simulink model "ESE4481_hw4_controls"  (R2021a)
settings: Solver=VariableStepAuto  StartTime=0.0  StopTime=10.0  RelTol=1e-3
values from neighbouring files (symbols this model uses):
  K_A = place(A_aileron, B_aileron, [-2,-4,-1])    [ESE4481_hw4_poleplacement.m]
  K_E = place(A_elevator, B_elevator, [-2,-4,-1])    [ESE4481_hw4_poleplacement.m]
  K_R = place(A_rudder, B_rudder, [-2,-4])    [ESE4481_hw4_poleplacement.m]
  K_T = place(A_throttle, B_throttle, [-2,-4])    [ESE4481_hw4_poleplacement.m]
undefined symbols (not defined in the file or in its folder): A_aileron, A_elevator, A_rudder, A_throttle, B_aileron, B_elevator, B_rudder, B_throttle, F_aileron, F_elevator, F_rudder, F_throttle
settings Model: Creator=Liza  LastModifiedBy=Liza

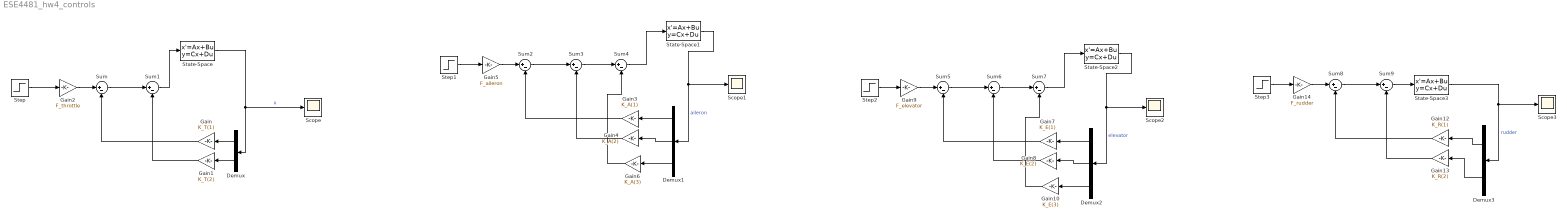
== system ESE4481_hw4_controls ==
  Demux : Demux  Outputs=2
  Demux1 : Demux  Outputs=3
  Demux2 : Demux  Outputs=3
  Demux3 : Demux  Outputs=2
  Gain : Gain  Gain=K_T(1)
  Gain1 : Gain  Gain=K_T(2)
  Gain10 : Gain  Gain=K_E(3)
  Gain12 : Gain  Gain=K_R(1)
  Gain13 : Gain  Gain=K_R(2)
  Gain14 : Gain  Gain=F_rudder
  Gain2 : Gain  Gain=F_throttle
  Gain3 : Gain  Gain=K_A(1)
  Gain4 : Gain  Gain=K_A(2)
  Gain5 : Gain  Gain=F_aileron
  Gain6 : Gain  Gain=K_A(3)
  Gain7 : Gain  Gain=K_E(1)
  Gain8 : Gain  Gain=K_E(2)
  Gain9 : Gain  Gain=F_elevator
  Scope{,1..3} (4 alike) : Scope
  State-Space : StateSpace  A=A_throttle  B=B_throttle  C=[1,0;0,1]  D=[0;0]  InitialCondition=[0,0]
  State-Space1 : StateSpace  A=A_aileron  B=B_aileron  C=[1,0,0;0,1,0;0,0,1]  D=[0;0;0]  InitialCondition=[0;0;0]
  State-Space2 : StateSpace  A=A_elevator  B=B_elevator  C=[1,0,0;0,1,0;0,0,1]  D=[0;0;0]  InitialCondition=[0;0;0]
  State-Space3 : StateSpace  A=A_rudder  B=B_rudder  C=[1,0;0,1]  D=[0;0]  InitialCondition=[0;0]
  Step : Step  Time=5  SampleTime=0
  Step1 : Step  Time=5  SampleTime=0
  Step2 : Step  Time=3  SampleTime=0
  Step3 : Step  Time=5  After=0  SampleTime=0
  Sum{,1..9} (10 alike) : Sum  Inputs=|+-
  wires:
  Sum/1 -> Sum1/1
  Sum1/1 -> State-Space/1
  State-Space/1 -> Demux/1, Scope/1  "x"
  Demux/1 -> Gain/1
  Demux/2 -> Gain1/1
  Gain1/1 -> Sum1/2
  Gain/1 -> Sum/2
  Gain2/1 -> Sum/1
  Step1/1 -> Gain5/1
  Gain4/1 -> Sum3/2
  Gain3/1 -> Sum2/2
  Demux1/2 -> Gain4/1
  Gain5/1 -> Sum2/1
  State-Space1/1 -> Demux1/1, Scope1/1  "aileron"
  Sum2/1 -> Sum3/1
  Demux1/1 -> Gain3/1
  Demux1/3 -> Gain6/1
  Sum3/1 -> Sum4/1
  Gain6/1 -> Sum4/2
  Sum4/1 -> State-Space1/1
  Sum7/1 -> State-Space2/1
  Step2/1 -> Gain9/1
  Demux2/3 -> Gain10/1
  Sum5/1 -> Sum6/1
  Gain8/1 -> Sum6/2
  Gain9/1 -> Sum5/1
  Demux2/2 -> Gain8/1
  State-Space2/1 -> Demux2/1, Scope2/1  "elevator"
  Demux2/1 -> Gain7/1
  Gain7/1 -> Sum5/2
  Sum6/1 -> Sum7/1
  Gain10/1 -> Sum7/2
  Step3/1 -> Gain14/1
  Gain14/1 -> Sum8/1
  Demux3/2 -> Gain13/1
  Gain13/1 -> Sum9/2
  Sum8/1 -> Sum9/1
  State-Space3/1 -> Demux3/1, Scope3/1  "rudder"
  Gain12/1 -> Sum8/2
  Demux3/1 -> Gain12/1
  Sum9/1 -> State-Space3/1
  Step/1 -> Gain2/1
